simulink model "VMC_14Dof_2024a"  (R2024a)
settings: Solver=FixedStepDiscrete  StartTime=0.0  StopTime=10.0  FixedStep=0.001  RelTol=1e-3
InitFcn:
  | unlinear_14DOF_Parameters
undefined symbols (not defined in the file): Bf, Br, Cp_fl, Cp_fr, Cp_rl, Cp_rr, Cs_f, eta_FMotor, eta_RMotor, f, g, He, Hp, i_fa, i_ra, i_sw, I_tire, Ix, Iy, Iz, ks_f, kw, Lf, Lr, m, mb, mu, mw, r, Sampletime, Standstill_buffer, vx0, vxlim, w0
libraries: simulink x32, slpidlib x6
(part 1 of 5)
settings Model: Creator=Technic  LastModifiedBy=Technic
settings SolverCC: ZeroCrossControl=EnableAll
settings OptimizationCC: DefaultParameterBehavior=Inlined  DefaultUnderspecifiedDataType=single  EnhancedBackFolding=on  PassReuseOutputArgsAs=Individual arguments  ZeroExternalMemoryAtStartup=off  ZeroInternalMemoryAtStartup=off  OptimizeBlockOrder=speed  DifferentSizesBufferReuse=on  OptimizationCustomize=off  EfficientTunableParamExpr=on
settings DebuggingCC: AlgebraicLoopMsg=error  BlockPriorityViolationMsg=error  SolverPrmCheckMsg=error  ParameterPrecisionLossMsg=none  ParamPrecisionLossAbsoluteDiffThreshold=1e-12  ParamPrecisionLossRelativeDiffThreshold=1e-10  ParameterTunabilityLossMsg=error  UnnecessaryDatatypeConvMsg=warning  StateNameClashWarn=warning  AllowedUnitSystems=SI,SI (extended)  AllowAutomaticUnitConversions=off
settings HardwareCC: ProdBitPerPointer=32  ProdBitPerSizeT=32  ProdBitPerPtrDiffT=32  ProdLargestAtomicInteger=Long  ProdLargestAtomicFloat=Double  ProdWordSize=32  ProdHWDeviceType=NXP->Cortex-M4
settings SFSimCC: MATLABDynamicMemAlloc=off
settings RTWCC: Description=Embedded Coder  SystemTargetFile=ert.tlc  GenCodeOnly=on  TemplateMakefile=ert_default_tmf  GenerateReport=on  LaunchReport=on
settings CodeAppCC: ForceParamTrailComments=on  IgnoreCustomStorageClasses=off  OperatorAnnotations=on  SimulinkDataObjDesc=on  SFDataObjDesc=on  InsertBlockDesc=on
settings ERTTargetCC: TargetLangStandard=C99 (ISO)  GenerateSampleERTMain=on  InlinedParameterPlacement=NonHierarchical  ERTCustomFileTemplate=example_file_process.tlc

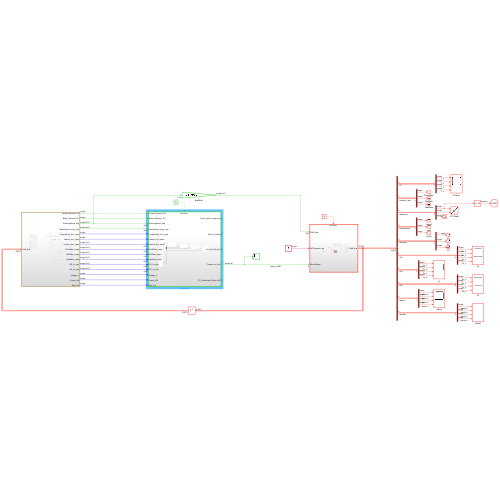
[thumbnail: Simulink's stored preview of the top-level diagram]
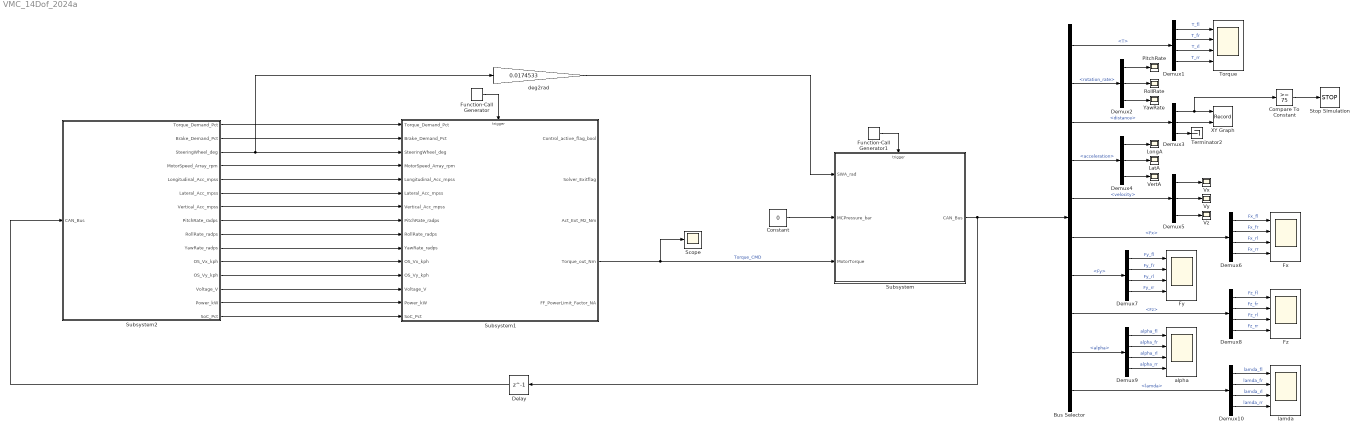
== system VMC_14Dof_2024a ==
  Bus Selector : BusSelector  OutputSignals=T,VehFdbk.rotation_rate,VehFdbk.distance,VehFdbk.acceleration,VehFdbk.velocity,Fx,Fy,Fz,alpha,lamda
  Compare To Constant : simulink/Logic and Bit Operations/Compare To Constant  relop=>=  const=75  OutDataTypeStr=boolean
  Constant : Constant  Value=0  OutDataTypeStr=single
  Delay : Delay  DelayLength=1  InputProcessing=Columns as channels (frame based)
  Demux{1,6..10} (6 alike) : Demux
  Demux{2..5} (4 alike) : Demux  Outputs=3
  Function-Call Generator : simulink/Ports & Subsystems/Function-Call Generator  sample_time=0.005  numberOfIterations=1  DisallowWideOutput=off
  Function-Call Generator1 : simulink/Ports & Subsystems/Function-Call Generator  sample_time=0.001  numberOfIterations=1  DisallowWideOutput=off
  Fx : Scope  NumInputPorts=4
  Fy : Scope  NumInputPorts=4
  Fz : Scope  NumInputPorts=4
  LatA : Scope
  LongA : Scope
  PitchRate : Scope
  RollRate : Scope
  Scope : Scope
  Stop Simulation : Stop
  Subsystem : Subsystem
  Subsystem1 : Subsystem
  Subsystem2 : Subsystem
  Terminator2 : Terminator
  Torque : Scope  NumInputPorts=4
  VertA : Scope
  Vx : Scope
  Vy : Scope
  Vz : Scope
  XY Graph : Record  FileSettingsInternal="{\"entries\":[{\"content\":{\"excelSettings\":{\"content\":{},\"type\":\"Streamout.ExcelSettings\"}},\"type\":\"Streamout.FileSettingStorage\",\"uuid\":\"\"}],\"packageUris\":[\"http:\\/\\/schema.mathworks.com\\/mf0\\/streamout_blocks\\/R2020a\"],\"version\":\"1.0\"}"  Layout=[1 1]  SignalsInternal="{\"entries\":[{\"content\":{\"signals\":[{\"content\":{\"blockPath\":[],\"dimensions\":[1],\"domain\":\"\",\"lineColor\":\"#a2142f\",\"plots\":[ 1 ],\"port\":1,\"signalID\":1,\"signalName\":\"Demux3:1\"},\"type\":\"RecordBlkView.Signal\",\"uuid\":\"\"},{\"content\":{\"blockPath\":[],\"dimensions\":[1],\"domain\":\"\",\"lineColor\":\"#139fff\",\"plots\":[ 1 ],\"port\":2,\"signalID\":2,\"signalName\":\"Demux3:2\"},\"type\":\"RecordBlkView.Signal\",\"uuid\":\"\"}]},\"type\":\"RecordBlkView.InputSignals\",\"uuid\":\"\"}],\"packageUris\":[\"http:\\/\\/schema.mathworks.com\\/mf0\\/streamout_blocks\\/R2020a\"],\"version\":\"1.0\"}"  VisualizationBindings="{\"xyplotplugin\":{\"info\":[{\"series\":[{\"bindingParametersList\":[{\"parameter\":\"X-Axis\",\"signalID\":1,\"signalName\":\"Demux3:1\"},{\"parameter\":\"Y-Axis\",\"signalID\":2,\"signalName\":\"Demux3:2\"}],\"seriesID\":0}],\"subplotID\":1}]}}"  CompatibilityTag=XY  st=-1
  YawRate : Scope
  alpha : Scope  NumInputPorts=4
  deg2rad : Gain  Gain=0.0174533
  lamda : Scope  NumInputPorts=4
  wires:
  Function-Call Generator/1 -> Subsystem1/Trigger
  Subsystem2/3(SteeringWheel_deg) -> deg2rad/1, Subsystem1/3(SteeringWheel_deg)
  Constant/1 -> Subsystem/2(MCPressure_bar)
  Subsystem1/4(Torque_out_Nm) -> Scope/1, Subsystem/3(MotorTorque)  "Torque_CMD"
  Function-Call Generator1/1 -> Subsystem/Trigger
  Subsystem2/1(Torque_Demand_Pct) -> Subsystem1/1(Torque_Demand_Pct)
  Subsystem2/2(Brake_Demand_Pct) -> Subsystem1/2(Brake_Demand_Pct)
  Subsystem2/4(MotorSpeed_Array_rpm) -> Subsystem1/4(MotorSpeed_Array_rpm)
  Subsystem2/5(Longitudinal_Acc_mpss) -> Subsystem1/5(Longitudinal_Acc_mpss)
  Subsystem2/6(Lateral_Acc_mpss) -> Subsystem1/6(Lateral_Acc_mpss)
  Subsystem2/7(Vertical_Acc_mpss) -> Subsystem1/7(Vertical_Acc_mpss)
  Subsystem2/8(PitchRate_radps) -> Subsystem1/8(PitchRate_radps)
  Subsystem2/9(RollRate_radps) -> Subsystem1/9(RollRate_radps)
  Subsystem2/10(YawRate_radps) -> Subsystem1/10(YawRate_radps)
  Subsystem2/11(OS_Vx_kph) -> Subsystem1/11(OS_Vx_kph)
  Subsystem2/12(OS_Vy_kph) -> Subsystem1/12(OS_Vy_kph)
  Subsystem2/13(Voltage_V) -> Subsystem1/13(Voltage_V)
  Subsystem2/14(Power_kW) -> Subsystem1/14(Power_kW)
  Subsystem2/15(SoC_Pct) -> Subsystem1/15(SoC_Pct)
  deg2rad/1 -> Subsystem/1(SWA_rad)
  Delay/1 -> Subsystem2/1(CAN_Bus)
  Demux8/2 -> Fz/2  "Fz_fr"
  Demux9/3 -> alpha/3  "alpha_rl"
  Demux1/3 -> Torque/3  "T_rl"
  Demux2/2 -> RollRate/1
  Demux6/4 -> Fx/4  "Fx_rr"
  Demux10/3 -> lamda/3  "lamda_rl"
  Demux4/3 -> VertA/1
  Demux7/2 -> Fy/2  "Fy_fr"
  Demux9/4 -> alpha/4  "alpha_rr"
  Bus Selector/9 -> Demux9/1  "<alpha>"
  Demux10/4 -> lamda/4  "lamda_rr"
  Demux8/4 -> Fz/4  "Fz_rr"
  Demux1/2 -> Torque/2  "T_fr"
  Demux5/3 -> Vz/1
  Demux4/2 -> LatA/1
  Bus Selector/7 -> Demux7/1  "<Fy>"
  Demux6/3 -> Fx/3  "Fx_rl"
  Demux3/3 -> Terminator2/1
  Bus Selector/4 -> Demux4/1  "<acceleration>"
  Bus Selector/6 -> Demux6/1  "<Fx>"
  Demux3/2 -> XY Graph/2
  Demux1/4 -> Torque/4  "T_rr"
  Bus Selector/3 -> Demux3/1  "<distance>"
  Demux9/2 -> alpha/2  "alpha_fr"
  Demux1/1 -> Torque/1  "T_fl"
  Demux8/3 -> Fz/3  "Fz_rl"
  Subsystem/1(CAN_Bus) -> Delay/1, Bus Selector/1
  Bus Selector/5 -> Demux5/1  "<velocity>"
  Demux8/1 -> Fz/1  "Fz_fl"
  Demux3/1 -> Compare To Constant/1, XY Graph/1
  Demux7/4 -> Fy/4  "Fy_rr"
  Demux5/1 -> Vx/1
  Compare To Constant/1 -> Stop Simulation/1
  Demux9/1 -> alpha/1  "alpha_fl"
  Bus Selector/10 -> Demux10/1  "<lamda>"
  Demux10/1 -> lamda/1  "lamda_fl"
  Demux7/1 -> Fy/1  "Fy_fl"
  Demux7/3 -> Fy/3  "Fy_rl"
  Demux5/2 -> Vy/1
  Demux2/1 -> PitchRate/1
  Demux6/1 -> Fx/1  "Fx_fl"
  Bus Selector/2 -> Demux2/1  "<rotation_rate>"
  Bus Selector/8 -> Demux8/1  "<Fz>"
  Demux10/2 -> lamda/2  "lamda_fr"
  Demux6/2 -> Fx/2  "Fx_fr"
  Demux2/3 -> YawRate/1
  Demux4/1 -> LongA/1
  Bus Selector/1 -> Demux1/1  "<T>"

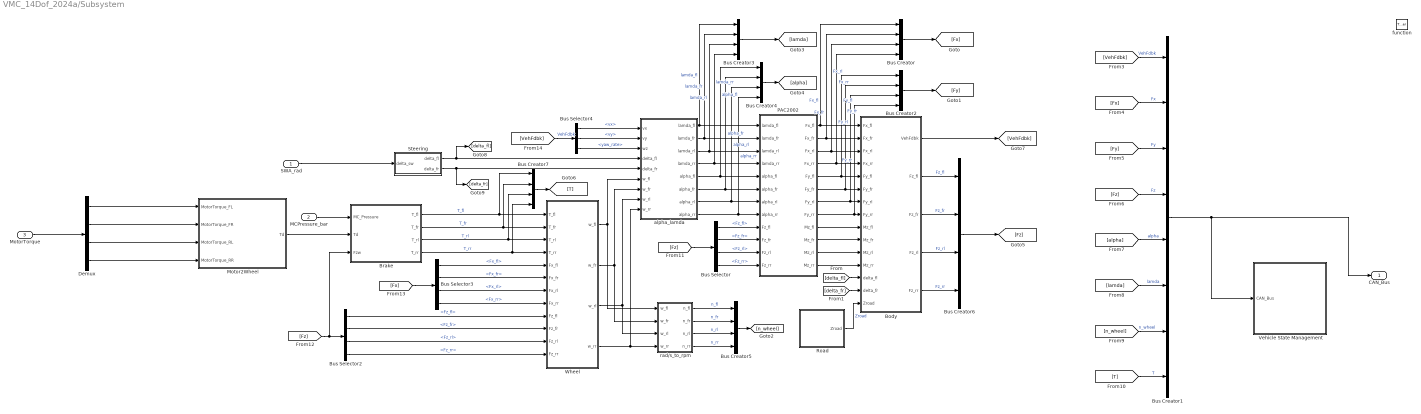
== system VMC_14Dof_2024a/Subsystem ==
  SWA_rad : Inport
  MCPressure_bar : Inport  Port=2
  MotorTorque : Inport  Port=3
  function : TriggerPort  TriggerType=function-call  VariantControl=(inherit)
  Body : Subsystem
  Brake : Subsystem
  Bus Creator{,2..7} (7 alike) : BusCreator  Inputs=4
  Bus Creator1 : BusCreator  Inputs=8
  Bus Selector : BusSelector  OutputSignals=Fz_fl,Fz_fr,Fz_rl,Fz_rr
  Bus Selector2 : BusSelector  OutputSignals=Fz_fl,Fz_fr,Fz_rl,Fz_rr
  Bus Selector3 : BusSelector  OutputSignals=Fx_fl,Fx_fr,Fx_rl,Fx_rr
  Bus Selector4 : BusSelector  OutputSignals=velocity.vx,velocity.vy,rotation_rate.yaw_rate
  Demux : Demux
  Motor2Wheel : Subsystem
  PAC2002 : Subsystem
  Road : Subsystem
  Steering : Subsystem
  Vehicle State Management : Subsystem
  Wheel : Subsystem
  alpha_lamda : Subsystem
  rad/s_to_rpm : Subsystem
  CAN_Bus : Outport  VectorParamsAs1DForOutWhenUnconnected=off
  wires:
  Demux/4 -> Motor2Wheel/4(MotorTorque_RR)
  Brake/2(T_fr) -> Wheel/2(T_fr), Bus Creator7/2  "T_fr"
  Brake/4(T_rr) -> Wheel/4(T_rr), Bus Creator7/4  "T_rr"
  PAC2002/9(Mz_fl) -> Body/9(Mz_fl)
  Bus Creator1/1 -> CAN_Bus/1, Vehicle State Management/1(CAN_Bus)
  Brake/3(T_rl) -> Wheel/3(T_rl), Bus Creator7/3  "T_rl"
  [VehFdbk] -> Bus Selector4/1  "VehFdbk"
  MCPressure_bar/1 -> Brake/1(MC_Pressure)
  [alpha] -> Bus Creator1/5  "alpha"
  Demux/3 -> Motor2Wheel/3(MotorTorque_RL)
  PAC2002/3(Fx_rl) -> Body/3(Fx_rl), Bus Creator/3  "Fx_rl"
  PAC2002/10(Mz_fr) -> Body/10(Mz_fr)
  Wheel/3(w_rl) -> alpha_lamda/8(w_rl), rad/s_to_rpm/3(w_rl)
  alpha_lamda/5(alpha_fl) -> Bus Creator4/1, PAC2002/5(alpha_fl)  "alpha_fl"
  Bus Creator3/1 -> [lamda]
  Bus Selector3/1 -> Wheel/5(Fx_fl)  "<Fx_fl>"
  Wheel/2(w_fr) -> alpha_lamda/7(w_fr), rad/s_to_rpm/2(w_fr)
  Steering/2(delta_fr) -> alpha_lamda/5(delta_fr), [delta_fr]
  Bus Selector2/1 -> Wheel/9(Fz_fl)  "<Fz_fl>"
  PAC2002/4(Fx_rr) -> Body/4(Fx_rr), Bus Creator/4  "Fx_rr"
  Bus Selector/2 -> PAC2002/10(Fz_fr)  "<Fz_fr>"
  Wheel/1(w_fl) -> alpha_lamda/6(w_fl), rad/s_to_rpm/1(w_fl)
  [Fx] -> Bus Selector3/1
  [T] -> Bus Creator1/8  "T"
  [Fz] -> Bus Creator1/4  "Fz"
  Body/2(Fz_fl) -> Bus Creator6/1  "Fz_fl"
  Bus Selector3/2 -> Wheel/6(Fx_fr)  "<Fx_fr>"
  Bus Selector2/3 -> Wheel/11(Fz_rl)  "<Fz_rl>"
  PAC2002/12(Mz_rr) -> Body/12(Mz_rr)
  Bus Creator2/1 -> [Fy]
  [VehFdbk] -> Bus Creator1/1  "VehFdbk"
  alpha_lamda/8(alpha_rr) -> Bus Creator4/4, PAC2002/8(alpha_rr)  "alpha_rr"
  PAC2002/2(Fx_fr) -> Body/2(Fx_fr), Bus Creator/2  "Fx_fr"
  Bus Selector2/2 -> Wheel/10(Fz_fr)  "<Fz_fr>"
  Bus Selector/4 -> PAC2002/12(Fz_rr)  "<Fz_rr>"
  [Fx] -> Bus Creator1/2  "Fx"
  rad/s_to_rpm/2(n_fr) -> Bus Creator5/2  "n_fr"
  Body/5(Fz_rr) -> Bus Creator6/4  "Fz_rr"
  alpha_lamda/3(lamda_rl) -> Bus Creator3/3, PAC2002/3(lamda_rl)  "lamda_rl"
  Bus Selector3/3 -> Wheel/7(Fx_rl)  "<Fx_rl>"
  Bus Selector/1 -> PAC2002/9(Fz_fl)  "<Fz_fl>"
  [n_wheel] -> Bus Creator1/7  "n_wheel"
  Bus Creator7/1 -> [T]
  [Fz] -> Brake/3(Fzw), Bus Selector2/1
  Body/3(Fz_fr) -> Bus Creator6/2  "Fz_fr"
  alpha_lamda/7(alpha_rl) -> Bus Creator4/3, PAC2002/7(alpha_rl)  "alpha_rl"
  [Fz] -> Bus Selector/1
  PAC2002/6(Fy_fr) -> Bus Creator2/2, Body/6(Fy_fr)  "Fy_fr"
  [delta_fl] -> Body/13(delta_fl)
  Bus Selector/3 -> PAC2002/11(Fz_rl)  "<Fz_rl>"
  Bus Selector3/4 -> Wheel/8(Fx_rr)  "<Fx_rr>"
  rad/s_to_rpm/4(n_rr) -> Bus Creator5/4  "n_rr"
  SWA_rad/1 -> Steering/1(delta_sw)
  Bus Selector4/3 -> alpha_lamda/3(wz)  "<yaw_rate>"
  [Fy] -> Bus Creator1/3  "Fy"
  MotorTorque/1 -> Demux/1
  alpha_lamda/1(lamda_fl) -> Bus Creator3/1, PAC2002/1(lamda_fl)  "lamda_fl"
  PAC2002/7(Fy_rl) -> Bus Creator2/3, Body/7(Fy_rl)  "Fy_rl"
  Road/1(Zroad) -> Body/15(Zroad)  "Zroad"
  [delta_fr] -> Body/14(delta_fr)
  Bus Creator6/1 -> [Fz]
  PAC2002/1(Fx_fl) -> Body/1(Fx_fl), Bus Creator/1  "Fx_fl"
  alpha_lamda/6(alpha_fr) -> Bus Creator4/2, PAC2002/6(alpha_fr)  "alpha_fr"
  Wheel/4(w_rr) -> alpha_lamda/9(w_rr), rad/s_to_rpm/4(w_rr)
  Motor2Wheel/1(Td) -> Brake/2(Td)
  Bus Creator4/1 -> [alpha]
  Bus Selector2/4 -> Wheel/12(Fz_rr)  "<Fz_rr>"
  alpha_lamda/2(lamda_fr) -> Bus Creator3/2, PAC2002/2(lamda_fr)  "lamda_fr"
  PAC2002/5(Fy_fl) -> Bus Creator2/1, Body/5(Fy_fl)  "Fy_fl"
  Demux/2 -> Motor2Wheel/2(MotorTorque_FR)
  Bus Creator5/1 -> [n_wheel]
  PAC2002/11(Mz_rl) -> Body/11(Mz_rl)
  Body/1(VehFdbk) -> [VehFdbk]
  alpha_lamda/4(lamda_rr) -> Bus Creator3/4, PAC2002/4(lamda_rr)  "lamda_rr"
  Bus Selector4/2 -> alpha_lamda/2(vy)  "<vy>"
  Demux/1 -> Motor2Wheel/1(MotorTorque_FL)
  PAC2002/8(Fy_rr) -> Bus Creator2/4, Body/8(Fy_rr)  "Fy_rr"
  rad/s_to_rpm/1(n_fl) -> Bus Creator5/1  "n_fl"
  rad/s_to_rpm/3(n_rl) -> Bus Creator5/3  "n_rl"
  Steering/1(delta_fl) -> alpha_lamda/4(delta_fl), [delta_fl]
  Bus Selector4/1 -> alpha_lamda/1(vx)  "<vx>"
  [lamda] -> Bus Creator1/6  "lamda"
  Bus Creator/1 -> [Fx]
  Brake/1(T_fl) -> Wheel/1(T_fl), Bus Creator7/1  "T_fl"
  Body/4(Fz_rl) -> Bus Creator6/3  "Fz_rl"

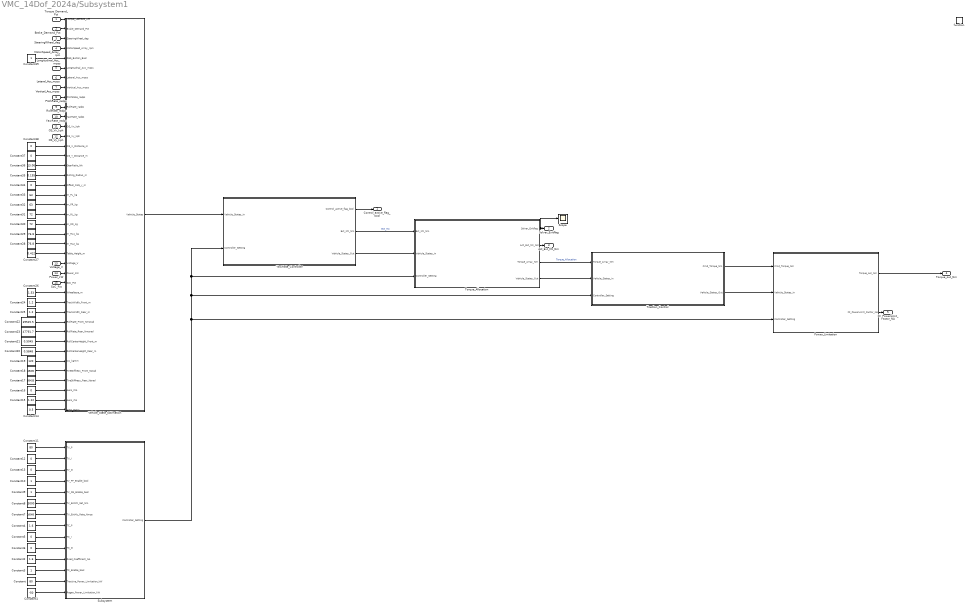
== system VMC_14Dof_2024a/Subsystem1 ==
  Torque_Demand_Pct : Inport
  Brake_Demand_Pct : Inport  Port=2
  SteeringWheel_deg : Inport  Port=3
  MotorSpeed_Array_rpm : Inport  Port=4
  Longitudinal_Acc_mpss : Inport  Port=5
  Lateral_Acc_mpss : Inport  Port=6
  Vertical_Acc_mpss : Inport  Port=7
  PitchRate_radps : Inport  Port=8
  RollRate_radps : Inport  Port=9
  YawRate_radps : Inport  Port=10
  OS_Vx_kph : Inport  Port=11
  OS_Vy_kph : Inport  Port=12
  Voltage_V : Inport  Port=13
  Power_kW : Inport  Port=14
  SoC_Pct : Inport  Port=15
  function : TriggerPort  TriggerType=function-call  VariantControl=(inherit)
  Constant : Constant  Value=80  OutDataTypeStr=single
  Constant1 : Constant  Value=-50  OutDataTypeStr=single
  Constant{3,9..10,39} (4 alike) : Constant  OutDataTypeStr=boolean
  Constant11 : Constant  Value=80  OutDataTypeStr=single
  Constant{5..6,12..13,16,34,37..38} (8 alike) : Constant  Value=0  OutDataTypeStr=single
  Constant14 : Constant  Value=0.5  OutDataTypeStr=single
  Constant15 : Constant  Value=1.22  OutDataTypeStr=single
  Constant17 : Constant  Value=50433  OutDataTypeStr=single
  Constant18 : Constant  Value=48482  OutDataTypeStr=single
  Constant19 : Constant  Value=120  OutDataTypeStr=single
  Constant2 : Constant  Value=1.6  OutDataTypeStr=single
  Constant20 : Constant  Value=0.5848  OutDataTypeStr=single
  Constant21 : Constant  Value=0.5045  OutDataTypeStr=single
  Constant22 : Constant  Value=39525.5  OutDataTypeStr=single
  Constant23 : Constant  Value=47791.7  OutDataTypeStr=single
  Constant24 : Constant  Value=1.2  OutDataTypeStr=single
  Constant25 : Constant  Value=1.2  OutDataTypeStr=single
  Constant26 : Constant  Value=1.53  OutDataTypeStr=single
  Constant27 : Constant  Value=0.412  OutDataTypeStr=single
  Constant28 : Constant  Value=76.8  OutDataTypeStr=single
  Constant29 : Constant  Value=76.8  OutDataTypeStr=single
  Constant30 : Constant  Value=72  OutDataTypeStr=single
  Constant31 : Constant  Value=72  OutDataTypeStr=single
  Constant32 : Constant  Value=63  OutDataTypeStr=single
  Constant33 : Constant  Value=63  OutDataTypeStr=single
  Constant35 : Constant  Value=0.195  OutDataTypeStr=single
  Constant36 : Constant  Value=13.06  OutDataTypeStr=single
  Constant4 : Constant  Value=1.6  OutDataTypeStr=single
  Constant7 : Constant  Value=10000  OutDataTypeStr=single
  Constant8 : Constant  Value=3000  OutDataTypeStr=single
  Power_Limitation : Subsystem
  Scope : Scope
  Subsystem : Subsystem
  Torque_Allocation : Subsystem  TreatAsAtomicUnit=on  RTWFcnName=Torque_Allocation
      settings: RTWSystemCode=Nonreusable function  RTWFcnNameOpts=User specified
  Traction_Control : Subsystem
  Vehicle_State_Estimation : Subsystem
  YawRate_Controller : Subsystem
  Control_active_flag_bool : Outport
  Solver_Exitflag : Outport  Port=2
  Act_Ext_Mz_Nm : Outport  Port=3
  Torque_out_Nm : Outport  Port=4
  FF_PowerLimit_Factor_NA : Outport  Port=5
  wires:
  Power_Limitation/2(FF_PowerLimit_Factor_NA) -> FF_PowerLimit_Factor_NA/1
  Constant36/1 -> Vehicle_State_Estimation/16(GearRatio_NA)
  Constant31/1 -> Vehicle_State_Estimation/21(m_RL_kg)
  Constant9/1 -> Subsystem/5(TV_FB_Enable_bool)
  Constant25/1 -> Vehicle_State_Estimation/31(TrackWidth_Rear_m)
  YawRate_radps/1 -> Vehicle_State_Estimation/11(YawRate_radps)
  Constant11/1 -> Subsystem/1(TV_P)
  Constant34/1 -> Vehicle_State_Estimation/18(Offset_CoG_y_m)
  Constant30/1 -> Vehicle_State_Estimation/22(m_RR_kg)
  Constant5/1 -> Subsystem/9(TC_I)
  YawRate_Controller/3(Vehicle_States_Out) -> Torque_Allocation/2(Vehicle_States_In)
  Constant1/1 -> Subsystem/14(Regen_Power_Limitation_kW)
  Constant7/1 -> Subsystem/7(TV_ExtMz_Rate_Nmps)
  Subsystem/1(Controller_Setting) -> Torque_Allocation/3(Controller_Setting), YawRate_Controller/2(Controller_Setting), Traction_Control/3(Controller_Setting), Power_Limitation/3(Controller_Setting)
  SteeringWheel_deg/1 -> Vehicle_State_Estimation/3(SteeringWheel_deg)
  Traction_Control/2(Vehicle_States_Out) -> Power_Limitation/2(Vehicle_States_In)
  Power_Limitation/1(Torque_out_Nm) -> Torque_out_Nm/1
  Constant35/1 -> Vehicle_State_Estimation/17(Rolling_Radius_m)
  RollRate_radps/1 -> Vehicle_State_Estimation/10(RollRate_radps)
  Constant10/1 -> Subsystem/4(TV_FF_Enable_bool)
  Constant6/1 -> Subsystem/10(TC_D)
  Lateral_Acc_mpss/1 -> Vehicle_State_Estimation/7(Lateral_Acc_mpss)
  PitchRate_radps/1 -> Vehicle_State_Estimation/9(PitchRate_radps)
  Torque_Allocation/3(Torque_Array_Nm) -> Traction_Control/1(Torque_Array_Nm)  "Torque_Allocation"
  Torque_Allocation/4(Vehicle_States_Out) -> Traction_Control/2(Vehicle_States_In)
  Constant28/1 -> Vehicle_State_Estimation/24(m_RL2_kg)
  Constant23/1 -> Vehicle_State_Estimation/33(RollRate_Rear_Nmprad)
  Longitudinal_Acc_mpss/1 -> Vehicle_State_Estimation/6(Longitudinal_Acc_mpss)
  Constant2/1 -> Subsystem/11(Road_Coefficient_NA)
  YawRate_Controller/2(Ext_Mz_Nm) -> Torque_Allocation/1(Ext_Mz_Nm)  "Ext_Mz"
  Constant38/1 -> Vehicle_State_Estimation/14(OS_X_Distance_m)
  MotorSpeed_Array_rpm/1 -> Vehicle_State_Estimation/4(MotorSpeed_Array_rpm)
  Constant26/1 -> Vehicle_State_Estimation/29(Wheelbase_m)
  Constant18/1 -> Vehicle_State_Estimation/37(TireStiffness_Front_Nprad)
  Constant22/1 -> Vehicle_State_Estimation/32(RollRate_Front_Nmprad)
  Traction_Control/1(Cmd_Torque_Nm) -> Power_Limitation/1(Cmd_Torque_Nm)
  Constant16/1 -> Vehicle_State_Estimation/39(Aero_ClA)
  OS_Vx_kph/1 -> Vehicle_State_Estimation/12(OS_Vx_kph)
  Constant12/1 -> Subsystem/2(TV_I)
  Brake_Demand_Pct/1 -> Vehicle_State_Estimation/2(Brake_Demand_Pct)
  Constant39/1 -> Vehicle_State_Estimation/5(REG_Button_Bool)
  Constant32/1 -> Vehicle_State_Estimation/20(m_FR_kg)
  Constant4/1 -> Subsystem/8(TC_P)
  Constant21/1 -> Vehicle_State_Estimation/34(RollCenterHeight_Front_m)
  Power_kW/1 -> Vehicle_State_Estimation/27(Power_kW)
  Constant13/1 -> Subsystem/3(TV_D)
  Constant27/1 -> Vehicle_State_Estimation/25(Table_Height_m)
  Constant33/1 -> Vehicle_State_Estimation/19(m_FL_kg)
  Torque_Demand_Pct/1 -> Vehicle_State_Estimation/1(Torque_Demand_Pct)
  Constant29/1 -> Vehicle_State_Estimation/23(m_RL1_kg)
  Constant3/1 -> Subsystem/12(TC_Enable_bool)
  Constant24/1 -> Vehicle_State_Estimation/30(TrackWidth_Front_m)
  Constant19/1 -> Vehicle_State_Estimation/36(Izz_kgmm)
  Constant20/1 -> Vehicle_State_Estimation/35(RollCenterHeight_Rear_m)
  Vehicle_State_Estimation/1(Vehicle_States) -> YawRate_Controller/1(Vehicle_States_In)
  Constant14/1 -> Vehicle_State_Estimation/41(Aero_Ratio)
  Constant/1 -> Subsystem/13(Tractive_Power_Limitation_kW)
  OS_Vy_kph/1 -> Vehicle_State_Estimation/13(OS_Vy_kph)
  Constant15/1 -> Vehicle_State_Estimation/40(Aero_rho)
  Constant17/1 -> Vehicle_State_Estimation/38(TireStiffness_Rear_Nprad)
  Constant37/1 -> Vehicle_State_Estimation/15(OS_Y_Distance_m)
  Constant8/1 -> Subsystem/6(TV_ExtMz_Sat_Nm)
  Vertical_Acc_mpss/1 -> Vehicle_State_Estimation/8(Vertical_Acc_mpss)
  Voltage_V/1 -> Vehicle_State_Estimation/26(Voltage_V)
  SoC_Pct/1 -> Vehicle_State_Estimation/28(SoC_Pct)
  Torque_Allocation/1(Solver_Exitflag) -> Scope/1, Solver_Exitflag/1
  YawRate_Controller/1(Control_active_flag_bool) -> Control_active_flag_bool/1
  Torque_Allocation/2(Act_Ext_Mz_Nm) -> Act_Ext_Mz_Nm/1

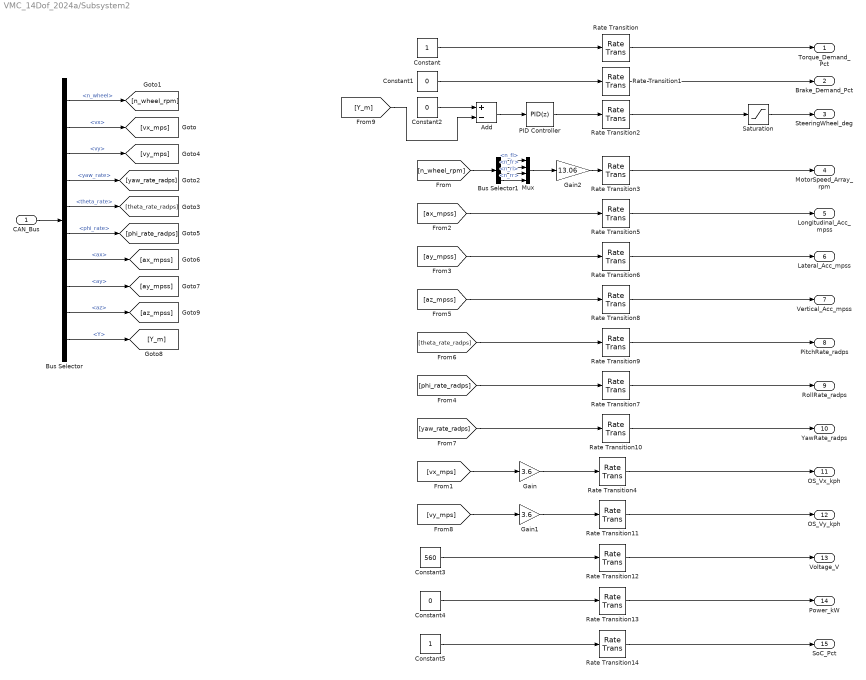
== system VMC_14Dof_2024a/Subsystem2 ==
  CAN_Bus : Inport
  Add : Sum  Inputs=+-
  Bus Selector : BusSelector  OutputSignals=n_wheel,VehFdbk.velocity.vx,VehFdbk.velocity.vy,VehFdbk.rotation_rate.yaw_rate,VehFdbk.rotation_rate.theta_rate,VehFdbk.rotation_rate.phi_rate,VehFdbk.acceleration.ax,VehFdbk.acceleration.ay,VehFdbk.acceleration.az,VehFdbk.distance.Y
  Bus Selector1 : BusSelector  OutputSignals=n_fl,n_fr,n_rl,n_rr
  Constant : Constant  OutDataTypeStr=single
  Constant1 : Constant  Value=0  OutDataTypeStr=single
  Constant2 : Constant  Value=0  OutDataTypeStr=single
  Constant3 : Constant  Value=560  OutDataTypeStr=single
  Constant4 : Constant  Value=0  OutDataTypeStr=single
  Constant5 : Constant  OutDataTypeStr=single
  Gain : Gain  Gain=3.6
  Gain1 : Gain  Gain=3.6
  Gain2 : Gain  Gain=13.06
  Mux : Mux
  PID Controller : slpidlib/PID Controller  Controller=PID  Form=Parallel  TimeDomain=Discrete-time  UseExternalTs=off  SampleTime=-1  IntegratorMethod=Forward Euler  FilterMethod=Forward Euler  ControllerParametersSource=internal  P=5  I=0  UseKiTs=off  D=50  UseExternalDerivativeSource=off  N=100  UseFilter=on  TunerSelectOption=Transfer Function Based (PID Tuner App)  InitialConditionSource=internal  InitialConditionForIntegrator=0  InitialConditionForFilter=0  DifferentiatorICPrevScaledInput=0  ExternalReset=none  TrackingMode=off  Kt=1  LimitOutput=off  SatLimitsSource=internal  UpperSaturationLimit=inf  LowerSaturationLimit=-inf  LinearizeAsGain=on  AntiWindupMode=none  Kb=1  LimitIntegrator=off  UpperIntegratorSaturationLimit=inf  LowerIntegratorSaturationLimit=-inf  POutMin=[]  POutMax=[]  IOutMin=[]  IOutMax=[]  DOutMin=[]  DOutMax=[]  NOutMin=[]  NOutMax=[]  SumOutMin=[]  SumOutMax=[]  SaturationOutMin=[]  SaturationOutMax=[]  PParamMin=[]  PParamMax=[]  IParamMin=[]  IParamMax=[]  DParamMin=[]  DParamMax=[]  NParamMin=[]  NParamMax=[]  KbParamMin=[]  KbParamMax=[]  KtParamMin=[]  KtParamMax=[]  KbOutMin=[]  KbOutMax=[]  KtOutMin=[]  KtOutMax=[]  IntegratorOutMin=[]  IntegratorOutMax=[]  FilterOutMin=[]  FilterOutMax=[]  SumI1OutMin=[]  SumI1OutMax=[]  SumI2OutMin=[]  SumI2OutMax=[]  SumI3OutMin=[]  SumI3OutMax=[]  SumI4OutMin=[]  SumI4OutMax=[]  SumDOutMin=[]  SumDOutMax=[]  DifferentiatorOutMin=[]  DifferentiatorOutMax=[]  FilterDiffOutCoefMin=[]  FilterDiffOutCoefMax=[]  ReciprocalOutMin=[]  ReciprocalOutMax=[]  SumDenOutMin=[]  SumDenOutMax=[]  SumNumOutMin=[]  SumNumOutMax=[]  DivideOutMin=[]  DivideOutMax=[]  UdiffTsProdOutMin=[]  UdiffTsProdOutMax=[]  NTsProdOutMin=[]  NTsProdOutMax=[]  UintegralTsProdOutMin=[]  UintegralTsProdOutMax=[]  UngainTsProdOutMin=[]  UngainTsProdOutMax=[]  ClampingZeroOutDataTypeStr=Inherit: Inherit via back propagation  ClampingZeroOutMin=[]  ClampingZeroOutMax=[]  FilterDenConstantOutDataTypeStr=Inherit: Inherit via back propagation  FilterDenConstantOutMin=[]  FilterDenConstantOutMax=[]  PCopyOutDataTypeStr=Inherit: Inherit via back propagation  PCopyOutMin=[]  PCopyOutMax=[]  NCopyOutDataTypeStr=Inherit: Inherit via back propagation  NCopyOutMin=[]  NCopyOutMax=[]  IntegratorContinuousStateAttributes=''  IntegratorStateMustResolveToSignalObject=off  IntegratorRTWStateStorageClass=Auto  FilterContinuousStateAttributes=''  FilterStateMustResolveToSignalObject=off  FilterRTWStateStorageClass=Auto  ParallelPVariant=InternalParameters  IdealPVariant=Disabled  IVariant=InternalParameters  DVariant=InternalParameters  IntegratorVariant=Discrete  SatVariant=Disabled  AWVariant=Passthrough  PCopyVariant=Disabled  TRVariant=Disabled  FdbkBlocksVariant=Forward  IdealPFdbkVariant=Disabled  SatFdbkVariant=Disabled  DerivativeFilterVariant=ForwardEulerFilter  NVariant=InternalParameters  NCopyVariant=Disabled  FilterICVariant=InternalICsFilter  IntegratorICVariant=InternalICs  ExternalResetVariant=Disabled  TRSumVariant=Passthrough  SumFdbkVariant=Disabled  SumVariant=Sum_PID  TsampFilterVariant=InternalTs  TsampNgainVariant=Passthrough  TsampIntegralVariant=Disabled_SignalSpec  ExternalSaturationOutDataTypeStr=Inherit: Same as second input  DerivativeSourceVariant=ErrorSignal
  Rate Transition{,1..3} (4 alike) : RateTransition  OutPortSampleTime=0.005
  Rate Transition{4..11} (8 alike) : RateTransition  OutPortSampleTime=0.02
  Rate Transition12 : RateTransition  OutPortSampleTime=0.01
  Rate Transition13 : RateTransition  OutPortSampleTime=0.01
  Rate Transition14 : RateTransition  OutPortSampleTime=0.01
  Saturation : Saturate  UpperLimit=117  LowerLimit=-117
  Torque_Demand_Pct : Outport
  Brake_Demand_Pct : Outport  Port=2
  SteeringWheel_deg : Outport  Port=3
  MotorSpeed_Array_rpm : Outport  Port=4
  Longitudinal_Acc_mpss : Outport  Port=5
  Lateral_Acc_mpss : Outport  Port=6
  Vertical_Acc_mpss : Outport  Port=7
  PitchRate_radps : Outport  Port=8
  RollRate_radps : Outport  Port=9
  YawRate_radps : Outport  Port=10
  OS_Vx_kph : Outport  Port=11
  OS_Vy_kph : Outport  Port=12
  Voltage_V : Outport  Port=13
  Power_kW : Outport  Port=14
  SoC_Pct : Outport  Port=15
  wires:
  Constant/1 -> Rate Transition/1
  Constant1/1 -> Rate Transition1/1
  Constant2/1 -> Add/1
  CAN_Bus/1 -> Bus Selector/1
  Bus Selector/10 -> [Y_m]  "<Y>"
  Bus Selector/2 -> [vx_mps]  "<vx>"
  Bus Selector/1 -> [n_wheel_rpm]  "<n_wheel>"
  Bus Selector/4 -> [yaw_rate_radps]  "<yaw_rate>"
  Bus Selector/5 -> [theta_rate_radps]  "<theta_rate>"
  Bus Selector/3 -> [vy_mps]  "<vy>"
  Bus Selector/6 -> [phi_rate_radps]  "<phi_rate>"
  Bus Selector/7 -> [ax_mpss]  "<ax>"
  Bus Selector/8 -> [ay_mpss]  "<ay>"
  Bus Selector1/1 -> Mux/1  "<n_fl>"
  Bus Selector1/2 -> Mux/2  "<n_fr>"
  Bus Selector1/3 -> Mux/3  "<n_rl>"
  Bus Selector1/4 -> Mux/4  "<n_rr>"
  Mux/1 -> Gain2/1
  Rate Transition3/1 -> MotorSpeed_Array_rpm/1
  [vx_mps] -> Gain/1
  Gain/1 -> Rate Transition4/1
  Rate Transition4/1 -> OS_Vx_kph/1
  [ax_mpss] -> Rate Transition5/1
  Rate Transition5/1 -> Longitudinal_Acc_mpss/1
  [ay_mpss] -> Rate Transition6/1
  Rate Transition6/1 -> Lateral_Acc_mpss/1
  Bus Selector/9 -> [az_mpss]  "<az>"
  [az_mpss] -> Rate Transition8/1
  Rate Transition8/1 -> Vertical_Acc_mpss/1
  [phi_rate_radps] -> Rate Transition7/1
  [theta_rate_radps] -> Rate Transition9/1
  Rate Transition9/1 -> PitchRate_radps/1
  Rate Transition7/1 -> RollRate_radps/1
  [yaw_rate_radps] -> Rate Transition10/1
  Rate Transition10/1 -> YawRate_radps/1
  Rate Transition11/1 -> OS_Vy_kph/1
  Gain1/1 -> Rate Transition11/1
  [vy_mps] -> Gain1/1
  Rate Transition12/1 -> Voltage_V/1
  Constant3/1 -> Rate Transition12/1
  Constant4/1 -> Rate Transition13/1
  Rate Transition13/1 -> Power_kW/1
  Rate Transition14/1 -> SoC_Pct/1
  Constant5/1 -> Rate Transition14/1
  Rate Transition/1 -> Torque_Demand_Pct/1
  Rate Transition1/1 -> Brake_Demand_Pct/1
  [Y_m] -> Add/2
  Add/1 -> PID Controller/1
  PID Controller/1 -> Rate Transition2/1
  Saturation/1 -> SteeringWheel_deg/1
  Rate Transition2/1 -> Saturation/1
  [n_wheel_rpm] -> Bus Selector1/1
  Gain2/1 -> Rate Transition3/1

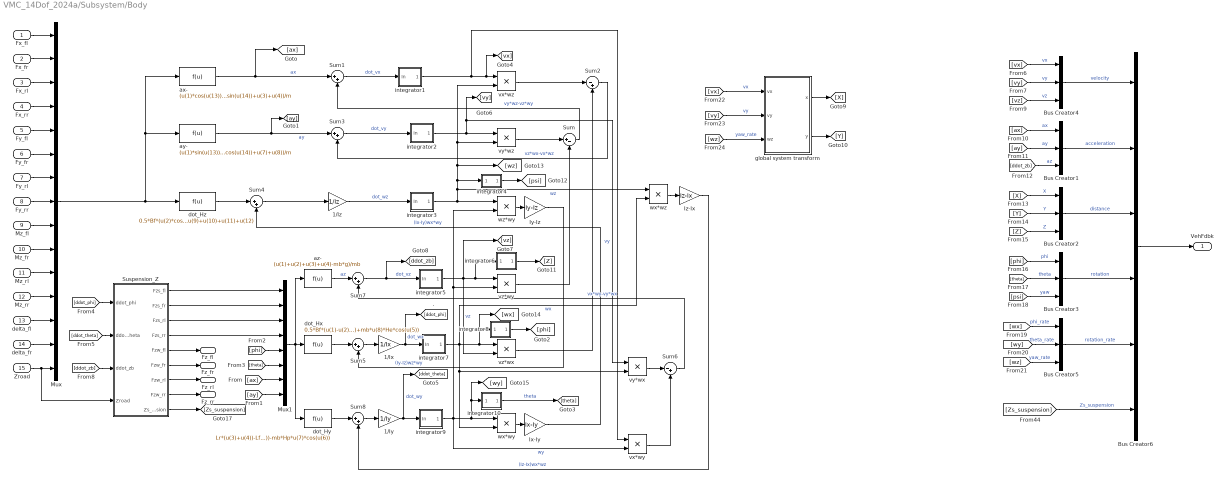
== system VMC_14Dof_2024a/Subsystem/Body ==
  Fx_fl : Inport
  Fx_fr : Inport  Port=2
  Fx_rl : Inport  Port=3
  Fx_rr : Inport  Port=4
  Fy_fl : Inport  Port=5
  Fy_fr : Inport  Port=6
  Fy_rl : Inport  Port=7
  Fy_rr : Inport  Port=8
  Mz_fl : Inport  Port=9
  Mz_fr : Inport  Port=10
  Mz_rl : Inport  Port=11
  Mz_rr : Inport  Port=12
  delta_fl : Inport  Port=13
  delta_fr : Inport  Port=14
  Zroad : Inport  Port=15
  1/Ix : Gain  Gain=1/Ix  OutDataTypeStr=single
  1/Iy : Gain  Gain=1/Iy  OutDataTypeStr=single
  1/Iz : Gain  Gain=1/Iz  OutDataTypeStr=single
  Bus Creator{1..5} (5 alike) : BusCreator  Inputs=3
  Bus Creator6 : BusCreator  Inputs=6
  Ix-Iy : Gain  Gain=Ix-Iy
  Iy-Iz : Gain  Gain=Iy-Iz
  Iz-Ix : Gain  Gain=Iz-Ix
  Mux : Mux  Inputs=15
  Mux1 : Mux  Inputs=8
  Sum : Sum  Inputs=|+-
  Sum1 : Sum  Inputs=|++  OutDataTypeStr=single  AccumDataTypeStr=single
  Sum2 : Sum  Inputs=|-+
  Sum{3..5,8} (4 alike) : Sum  Inputs=|++
  Sum6 : Sum  Inputs=|-+
  Sum7 : Sum  Inputs=|++  OutDataTypeStr=single
  Suspension_Z : Subsystem
  ax- : Fcn  Expr=(u(1)*cos(u(13))+u(2)*cos(u(14))-u(5)*sin(u(13))-u(6)*sin(u(14))+u(3)+u(4))/m
  ay- : Fcn  Expr=(u(1)*sin(u(13))+u(2)*sin(u(14))+u(5)*cos(u(13))+u(6)*cos(u(14))+u(7)+u(8))/m
  az- : Fcn  Expr=(u(1)+u(2)+u(3)+u(4)-mb*g)/mb
  dot_Hx : Fcn  Expr=0.5*Bf*(u(1)-u(2))+0.5*Br*(u(3)-u(4))+mb*g*He*sin(u(5))+mb*u(8)*He*cos(u(5))
  dot_Hy : Fcn  Expr=Lr*(u(3)+u(4))-Lf*(u(1)+u(2))+mb*g*Hp*sin(u(6))-mb*Hp*u(7)*cos(u(6))
  dot_Hz : Fcn  Expr=0.5*Bf*(u(2)*cos(u(14))-u(1)*cos(u(13))-u(6)*sin(u(14))+u(5)*sin(u(13)))+0.5*Br*(u(4)-u(3))+Lf*(u(1)*sin(u(13))+u(5)*cos(u(13))+u(2)*sin(u(14))+u(6)*cos(u(14)))-Lr*(u(7)+u(8))+u(9)+u(10)+u(11)+u(12)
  global system transform : Subsystem
  integrator1 : Subsystem
  integrator10 : Subsystem
  integrator2 : Subsystem
  integrator3 : Subsystem
  integrator4 : Subsystem
  integrator5 : Subsystem
  integrator6 : Subsystem
  integrator7 : Subsystem
  integrator8 : Subsystem
  integrator9 : Subsystem
  vx*wy : Product
  vx*wz : Product
  vy*wx : Product
  vy*wz : Product
  vz*wx : Product
  vz*wy : Product
  wx*wy : Product
  wx*wz : Product
  wz*wy : Product
  VehFdbk : Outport  VectorParamsAs1DForOutWhenUnconnected=off
  Fz_fl : Outport  Port=2  VectorParamsAs1DForOutWhenUnconnected=off
  Fz_fr : Outport  Port=3  VectorParamsAs1DForOutWhenUnconnected=off
  Fz_rl : Outport  Port=4  VectorParamsAs1DForOutWhenUnconnected=off
  Fz_rr : Outport  Port=5  VectorParamsAs1DForOutWhenUnconnected=off
  wires:
  Mux1/1 -> az-/1, dot_Hx/1, dot_Hy/1
  Sum8/1 -> 1/Iy/1
  az-/1 -> Sum7/1  "az"
  dot_Hy/1 -> Sum8/1
  ax-/1 -> [ax], Sum1/1  "ax"
  Suspension_Z/8(Fzw_rr) -> Fz_rr/1
  Suspension_Z/7(Fzw_rl) -> Fz_rl/1
  Suspension_Z/6(Fzw_fr) -> Fz_fr/1
  Suspension_Z/5(Fzw_fl) -> Fz_fl/1
  [ddot_zb] -> Suspension_Z/3(ddot_zb)
  [ddot_theta] -> Suspension_Z/2(ddot_theta)
  [ddot_phi] -> Suspension_Z/1(ddot_phi)
  [phi] -> Mux1/5
  Suspension_Z/2(Fzs_fr) -> Mux1/2
  Suspension_Z/3(Fzs_rl) -> Mux1/3
  Suspension_Z/4(Fzs_rr) -> Mux1/4
  Suspension_Z/1(Fzs_fl) -> Mux1/1
  integrator10/1(Out) -> [theta]  "theta"
  Iz-Ix/1 -> Sum8/2  "(Iz-Ix)wx*wz"
  wx*wz/1 -> Iz-Ix/1
  Sum5/1 -> 1/Ix/1
  Iy-Iz/1 -> Sum5/2  "(Iy-Iz)wz*wy"
  dot_Hx/1 -> Sum5/1
  Sum6/1 -> Sum7/2  "vx*wy-vy*wx"
  vx*wy/1 -> Sum6/2
  vy*wx/1 -> Sum6/1
  Sum4/1 -> 1/Iz/1
  dot_Hz/1 -> Sum4/1
  Ix-Iy/1 -> Sum4/2  "(Ix-Iy)wx*wy"
  wx*wy/1 -> Ix-Iy/1
  Sum2/1 -> Sum3/2  "vz*wx-vx*wz"
  vz*wx/1 -> Sum2/2
  vx*wz/1 -> Sum2/1
  Sum/1 -> Sum1/2  "vy*wz-vz*wy"
  vz*wy/1 -> Sum/2
  wz*wy/1 -> Iy-Iz/1
  vy*wz/1 -> Sum/1
  ay-/1 -> [ay], Sum3/1  "ay"
  integrator9/1(Out) -> wx*wy/1, integrator10/1(In), [wy], wz*wy/2, vz*wy/2, vx*wy/2  "wy"
  1/Iy/1 -> integrator9/1(In), [ddot_theta]  "dot_wy"
  1/Ix/1 -> integrator7/1(In), [ddot_phi]  "dot_wx"
  integrator7/1(Out) -> integrator8/1(In), [wx], vz*wx/1, wx*wy/2, vy*wx/2, wx*wz/2  "wx"
  integrator5/1(Out) -> [vz], integrator6/1(In), vz*wy/1, vz*wx/2  "vz"
  Sum7/1 -> integrator5/1(In), [ddot_zb]  "dot_vz"
  integrator3/1(Out) -> wz*wy/1, [wz], vx*wz/2, vy*wz/2, integrator4/1(In), wx*wz/1  "wz"
  1/Iz/1 -> integrator3/1(In)  "dot_wz"
  Sum3/1 -> integrator2/1(In)  "dot_vy"
  integrator2/1(Out) -> vy*wz/1, [vy], vy*wx/1  "vy"
  integrator1/1(Out) -> vx*wy/1, [vx], vx*wz/1
  Sum1/1 -> integrator1/1(In)  "dot_vx"
  Fx_fl/1 -> Mux/1
  Fx_fr/1 -> Mux/2
  Fx_rl/1 -> Mux/3
  Fx_rr/1 -> Mux/4
  Fy_fl/1 -> Mux/5
  Fy_fr/1 -> Mux/6
  Fy_rl/1 -> Mux/7
  Fy_rr/1 -> Mux/8
  Mz_fl/1 -> Mux/9
  Mz_fr/1 -> Mux/10
  Mz_rl/1 -> Mux/11
  Mz_rr/1 -> Mux/12
  delta_fl/1 -> Mux/13
  delta_fr/1 -> Mux/14
  Mux/1 -> ax-/1, ay-/1, dot_Hz/1
  Zroad/1 -> Suspension_Z/4(Zroad), Mux/15
  [ax] -> Mux1/7
  [ay] -> Mux1/8
  global system transform/1(x) -> [X]
  global system transform/2(y) -> [Y]
  [theta] -> Mux1/6
  [ax] -> Bus Creator1/1  "ax"
  Bus Creator2/1 -> Bus Creator6/3  "distance"
  Bus Creator6/1 -> VehFdbk/1
  Bus Creator5/1 -> Bus Creator6/5  "rotation_rate"
  Bus Creator3/1 -> Bus Creator6/4  "rotation"
  [Y] -> Bus Creator2/2  "Y"
  [Zs_suspension] -> Bus Creator6/6  "Zs_suspension"
  [theta] -> Bus Creator3/2  "theta"
  [wz] -> Bus Creator5/3  "yaw_rate"
  [vx] -> Bus Creator4/1  "vx"
  [vy] -> Bus Creator4/2  "vy"
  [ay] -> Bus Creator1/2  "ay"
  [wy] -> Bus Creator5/2  "theta_rate"
  [ddot_zb] -> Bus Creator1/3  "az"
  [Z] -> Bus Creator2/3  "Z"
  Bus Creator4/1 -> Bus Creator6/1  "velocity"
  [phi] -> Bus Creator3/1  "phi"
  [vz] -> Bus Creator4/3  "vz"
  Bus Creator1/1 -> Bus Creator6/2  "acceleration"
  [wx] -> Bus Creator5/1  "phi_rate"
  [psi] -> Bus Creator3/3  "yaw"
  [X] -> Bus Creator2/1  "X"
  integrator6/1(Out) -> [Z]
  integrator4/1(Out) -> [psi]
  [vx] -> global system transform/1(vx)  "vx"
  [vy] -> global system transform/2(vy)  "vy"
  Suspension_Z/9(Zs_suspension) -> [Zs_suspension]
  [wz] -> global system transform/3(wz)  "yaw_rate"
  integrator8/1(Out) -> [phi]

== system VMC_14Dof_2024a/Subsystem/Brake ==
  MC_Pressure : Inport
  Td : Inport  Port=2
  Fzw : Inport  Port=3
  Add{,1..3} (4 alike) : Sum  Inputs=+-  OutDataTypeStr=single
  Bus Selector1 : BusSelector  OutputSignals=T_fl,T_fr,T_rl,T_rr
  Bus Selector3 : BusSelector  OutputSignals=Tb_fl,Tb_fr,Tb_rl,Tb_rr
  WheelBrakeTorque : Subsystem
  T_fl : Outport
  T_fr : Outport  Port=2
  T_rl : Outport  Port=3
  T_rr : Outport  Port=4
  wires:
  Bus Selector3/2 -> [Tb_fr]  "<Tb_fr>"
  Fzw/1 -> WheelBrakeTorque/3(Fzw)
  Add1/1 -> T_fr/1
  Bus Selector1/2 -> [Td_fr]  "<T_fr>"
  Bus Selector3/3 -> [Tb_rl]  "<Tb_rl>"
  [Tb_fl] -> Add/2  "Tb_fl"
  Bus Selector1/3 -> [Td_rl]  "<T_rl>"
  [Tb_rl] -> Add2/2  "Tb_rl"
  Bus Selector3/1 -> [Tb_fl]  "<Tb_fl>"
  Bus Selector3/4 -> [Tb_rr]  "<Tb_rr>"
  Bus Selector1/1 -> [Td_fl]  "<T_fl>"
  [Tb_rr] -> Add3/2  "Tb_rr"
  Td/1 -> Bus Selector1/1, WheelBrakeTorque/2(Td)
  MC_Pressure/1 -> WheelBrakeTorque/1(TMC)
  Add/1 -> T_fl/1
  WheelBrakeTorque/1(WheelBrakeTorque) -> Bus Selector3/1
  [Td_rl] -> Add2/1
  Bus Selector1/4 -> [Td_rr]  "<T_rr>"
  [Td_rr] -> Add3/1
  Add3/1 -> T_rr/1
  [Td_fr] -> Add1/1
  Add2/1 -> T_rl/1
  [Td_fl] -> Add/1
  [Tb_fr] -> Add1/2  "Tb_fr"

== system VMC_14Dof_2024a/Subsystem/Motor2Wheel ==
  MotorTorque_FL : Inport
  MotorTorque_FR : Inport  Port=2
  MotorTorque_RL : Inport  Port=3
  MotorTorque_RR : Inport  Port=4
  Bus Creator : BusCreator  Inputs=4
  Gain : Gain  Gain=eta_FMotor  OutDataTypeStr=single
  Gain1 : Gain  Gain=eta_RMotor  ParamDataTypeStr=single  OutDataTypeStr=single
  Gain2 : Gain  Gain=i_ra  OutDataTypeStr=single
  Gain3 : Gain  Gain=i_ra  OutDataTypeStr=single
  Gain4 : Gain  Gain=eta_FMotor  OutDataTypeStr=single
  Gain5 : Gain  Gain=i_fa  OutDataTypeStr=single
  Gain6 : Gain  Gain=eta_FMotor  OutDataTypeStr=single
  Gain7 : Gain  Gain=i_fa  OutDataTypeStr=single
  Td : Outport  VectorParamsAs1DForOutWhenUnconnected=off
  wires:
  Gain7/1 -> [Td_fr]  "T_fr"
  Gain5/1 -> [Td_fl]  "T_fl"
  MotorTorque_FL/1 -> Gain/1
  Gain3/1 -> [Td_rr]  "T_rr"
  Gain2/1 -> [Td_rl]  "T_rl"
  MotorTorque_RL/1 -> Gain1/1
  [Td_rr] -> Bus Creator/4
  Bus Creator/1 -> Td/1
  [Td_rl] -> Bus Creator/3
  [Td_fl] -> Bus Creator/1
  [Td_fr] -> Bus Creator/2
  Gain/1 -> Gain5/1
  Gain1/1 -> Gain2/1
  MotorTorque_FR/1 -> Gain4/1
  MotorTorque_RR/1 -> Gain6/1
  Gain6/1 -> Gain3/1
  Gain4/1 -> Gain7/1

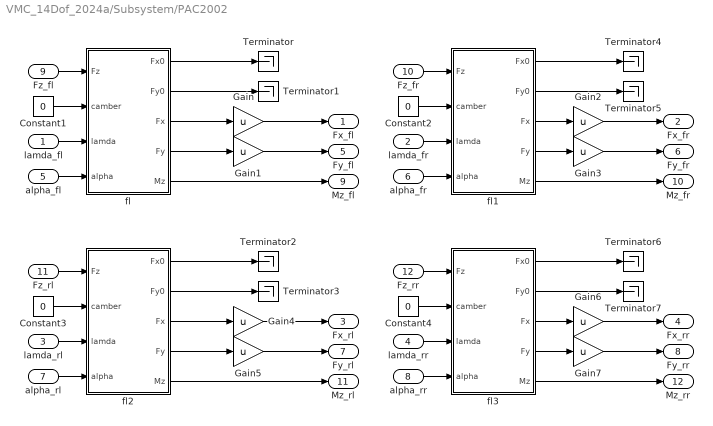
== system VMC_14Dof_2024a/Subsystem/PAC2002 ==
  lamda_fl : Inport
  lamda_fr : Inport  Port=2
  lamda_rl : Inport  Port=3
  lamda_rr : Inport  Port=4
  alpha_fl : Inport  Port=5
  alpha_fr : Inport  Port=6
  alpha_rl : Inport  Port=7
  alpha_rr : Inport  Port=8
  Fz_fl : Inport  Port=9
  Fz_fr : Inport  Port=10
  Fz_rl : Inport  Port=11
  Fz_rr : Inport  Port=12
  Constant{1..4} (4 alike) : Constant  Value=0  OutDataTypeStr=single
  Gain{,1..7} (8 alike) : Gain  Gain=u
  Terminator{,1..7} (8 alike) : Terminator
  fl : MATLAB Function  TreatAsAtomicUnit=on
  fl1 : MATLAB Function  TreatAsAtomicUnit=on
  fl2 : MATLAB Function  TreatAsAtomicUnit=on
  fl3 : MATLAB Function  TreatAsAtomicUnit=on
  Fx_fl : Outport  VectorParamsAs1DForOutWhenUnconnected=off
  Fx_fr : Outport  Port=2  VectorParamsAs1DForOutWhenUnconnected=off
  Fx_rl : Outport  Port=3  VectorParamsAs1DForOutWhenUnconnected=off
  Fx_rr : Outport  Port=4  VectorParamsAs1DForOutWhenUnconnected=off
  Fy_fl : Outport  Port=5  VectorParamsAs1DForOutWhenUnconnected=off
  Fy_fr : Outport  Port=6  VectorParamsAs1DForOutWhenUnconnected=off
  Fy_rl : Outport  Port=7  VectorParamsAs1DForOutWhenUnconnected=off
  Fy_rr : Outport  Port=8  VectorParamsAs1DForOutWhenUnconnected=off
  Mz_fl : Outport  Port=9  VectorParamsAs1DForOutWhenUnconnected=off
  Mz_fr : Outport  Port=10  VectorParamsAs1DForOutWhenUnconnected=off
  Mz_rl : Outport  Port=11  VectorParamsAs1DForOutWhenUnconnected=off
  Mz_rr : Outport  Port=12  VectorParamsAs1DForOutWhenUnconnected=off
  wires:
  Constant4/1 -> fl3/2(camber)
  Constant3/1 -> fl2/2(camber)
  Constant2/1 -> fl1/2(camber)
  Fz_rr/1 -> fl3/1(Fz)
  alpha_rr/1 -> fl3/4(alpha)
  lamda_rr/1 -> fl3/3(lamda)
  Fz_rl/1 -> fl2/1(Fz)
  alpha_rl/1 -> fl2/4(alpha)
  lamda_rl/1 -> fl2/3(lamda)
  Fz_fr/1 -> fl1/1(Fz)
  alpha_fr/1 -> fl1/4(alpha)
  lamda_fr/1 -> fl1/3(lamda)
  Constant1/1 -> fl/2(camber)
  Fz_fl/1 -> fl/1(Fz)
  alpha_fl/1 -> fl/4(alpha)
  lamda_fl/1 -> fl/3(lamda)
  fl/3(Fx) -> Gain/1
  fl/4(Fy) -> Gain1/1
  fl1/4(Fy) -> Gain3/1
  fl3/3(Fx) -> Gain6/1
  fl3/4(Fy) -> Gain7/1
  fl2/3(Fx) -> Gain4/1
  fl2/4(Fy) -> Gain5/1
  fl1/3(Fx) -> Gain2/1
  Gain/1 -> Fx_fl/1
  Gain1/1 -> Fy_fl/1
  Gain2/1 -> Fx_fr/1
  Gain3/1 -> Fy_fr/1
  Gain4/1 -> Fx_rl/1
  Gain5/1 -> Fy_rl/1
  Gain6/1 -> Fx_rr/1
  Gain7/1 -> Fy_rr/1
  fl/1(Fx0) -> Terminator/1
  fl/2(Fy0) -> Terminator1/1
  fl2/1(Fx0) -> Terminator2/1
  fl2/2(Fy0) -> Terminator3/1
  fl1/1(Fx0) -> Terminator4/1
  fl1/2(Fy0) -> Terminator5/1
  fl3/1(Fx0) -> Terminator6/1
  fl3/2(Fy0) -> Terminator7/1
  fl/5(Mz) -> Mz_fl/1
  fl2/5(Mz) -> Mz_rl/1
  fl1/5(Mz) -> Mz_fr/1
  fl3/5(Mz) -> Mz_rr/1

== system VMC_14Dof_2024a/Subsystem/Road ==
  Bus Creator : BusCreator  Inputs=4
  Constant{1..4} (4 alike) : Constant  Value=0  OutDataTypeStr=single
  Zroad : Outport  VectorParamsAs1DForOutWhenUnconnected=off
  wires:
  Constant3/1 -> Bus Creator/4  "Zroad_rr"
  Constant1/1 -> Bus Creator/2  "Zroad_fr"
  Constant2/1 -> Bus Creator/3  "Zroad_rl"
  Bus Creator/1 -> Zroad/1  "Zroad"
  Constant4/1 -> Bus Creator/1  "Zroad_fl"

== system VMC_14Dof_2024a/Subsystem/Steering ==
  delta_sw : Inport
  Add : Sum  OutDataTypeStr=single
  Add2 : Sum  Inputs=-+  OutDataTypeStr=single
  Add3 : Sum  OutDataTypeStr=single
  Constant : Constant  Value=Lr  OutDataTypeStr=single
  Constant1 : Constant  Value=Lf  OutDataTypeStr=single
  Constant2 : Constant  Value=i_sw  OutDataTypeStr=single
  Constant3 : Constant  Value=Br  OutDataTypeStr=single
  Divide : Product  Inputs=*/
  Divide1 : Product  Inputs=/*  OutDataTypeStr=single
  Divide2 : Product  Inputs=/*  OutDataTypeStr=single
  Gain : Gain  Gain=2
  Product : Product  OutDataTypeStr=single
  Product1 : Product
  Trigonometric Function : Trigonometry  Operator=atan
  Trigonometric Function1 : Trigonometry  Operator=tan
  Trigonometric Function2 : Trigonometry  Operator=atan
  delta_fl : Outport  VectorParamsAs1DForOutWhenUnconnected=off
  delta_fr : Outport  Port=2  VectorParamsAs1DForOutWhenUnconnected=off
  wires:
  Constant1/1 -> Add/1
  Constant/1 -> Add/2
  Add/1 -> Gain/1
  delta_sw/1 -> Divide/1
  Constant2/1 -> Divide/2
  Divide/1 -> Trigonometric Function1/1  "delta_s"
  Trigonometric Function1/1 -> Product/1, Product1/2
  Gain/1 -> Product/2, Add3/2, Add2/2
  Constant3/1 -> Product1/1
  Product1/1 -> Add3/1, Add2/1
  Add2/1 -> Divide1/1
  Product/1 -> Divide2/2, Divide1/2
  Divide1/1 -> Trigonometric Function/1
  Trigonometric Function/1 -> delta_fl/1
  Add3/1 -> Divide2/1
  Divide2/1 -> Trigonometric Function2/1
  Trigonometric Function2/1 -> delta_fr/1

== system VMC_14Dof_2024a/Subsystem/Vehicle State Management ==
  CAN_Bus : Inport
  Abs{,1..4} (5 alike) : Abs  SaturateOnIntegerOverflow=off
  Bus Selector : BusSelector  OutputSignals=n_wheel.n_fl,n_wheel.n_fr,n_wheel.n_rl,n_wheel.n_rr,VehFdbk.velocity.vx
  Gain{,1..3} (4 alike) : Gain  Gain=pi/30
  Logical Operator : Logic  Inputs=4  AllPortsSameDT=off  OutDataTypeStr=boolean
  Logical Operator1 : Logic  AllPortsSameDT=off  OutDataTypeStr=boolean
  StandStill_thres : Subsystem
  StandStill_thres1 : Subsystem
  StandStill_thres2 : Subsystem
  StandStill_thres3 : Subsystem
  StandStill_thres4 : Subsystem
  tag scope: StandStill_flag=global
  wires:
  Bus Selector/2 -> Abs1/1  "<n_fr>"
  Bus Selector/1 -> Abs/1  "<n_fl>"
  CAN_Bus/1 -> Bus Selector/1
  Bus Selector/4 -> Abs3/1  "<n_rr>"
  Bus Selector/3 -> Abs2/1  "<n_rl>"
  Abs/1 -> Gain/1
  Abs1/1 -> Gain1/1
  Abs2/1 -> Gain2/1
  Abs3/1 -> Gain3/1
  StandStill_thres/1(Out1) -> Logical Operator/1
  StandStill_thres1/1(Out1) -> Logical Operator/2
  StandStill_thres2/1(Out1) -> Logical Operator/3
  Abs4/1 -> StandStill_thres4/1(In1)
  Logical Operator/1 -> Logical Operator1/1
  StandStill_thres4/1(Out1) -> Logical Operator1/2
  Bus Selector/5 -> Abs4/1  "<vx>"
  Gain/1 -> StandStill_thres/1(In1)
  Gain1/1 -> StandStill_thres1/1(In1)
  Gain2/1 -> StandStill_thres2/1(In1)
  Logical Operator1/1 -> [StandStill_flag]
  StandStill_thres3/1(Out1) -> Logical Operator/4
  Gain3/1 -> StandStill_thres3/1(In1)

== system VMC_14Dof_2024a/Subsystem/Wheel ==
  T_fl : Inport
  T_fr : Inport  Port=2
  T_rl : Inport  Port=3
  T_rr : Inport  Port=4
  Fx_fl : Inport  Port=5
  Fx_fr : Inport  Port=6
  Fx_rl : Inport  Port=7
  Fx_rr : Inport  Port=8
  Fz_fl : Inport  Port=9
  Fz_fr : Inport  Port=10
  Fz_rl : Inport  Port=11
  Fz_rr : Inport  Port=12
  fl : Subsystem
  fr : Subsystem
  rl : Subsystem
  rr : Subsystem
  w_fl : Outport  VectorParamsAs1DForOutWhenUnconnected=off
  w_fr : Outport  Port=2  VectorParamsAs1DForOutWhenUnconnected=off
  w_rl : Outport  Port=3  VectorParamsAs1DForOutWhenUnconnected=off
  w_rr : Outport  Port=4  VectorParamsAs1DForOutWhenUnconnected=off
  wires:
  rr/1(w_rr) -> w_rr/1
  Fz_rr/1 -> rr/3(Fz_rr)
  Fx_rr/1 -> rr/2(Fx_rr)
  T_rr/1 -> rr/1(T_rr)
  rl/1(w_rl) -> w_rl/1
  Fz_rl/1 -> rl/3(Fz_rl)
  Fx_rl/1 -> rl/2(Fx_rl)
  T_rl/1 -> rl/1(T_rl)
  Fz_fr/1 -> fr/3(Fz_fr)
  Fx_fr/1 -> fr/2(Fx_fr)
  T_fr/1 -> fr/1(T_fr)
  fr/1(w_fr) -> w_fr/1
  fl/1(w_fl) -> w_fl/1
  Fz_fl/1 -> fl/3(Fz_fl)
  Fx_fl/1 -> fl/2(Fx_fl)
  T_fl/1 -> fl/1(T_fl)

== system VMC_14Dof_2024a/Subsystem/alpha_lamda ==
  vx : Inport
  vy : Inport  Port=2
  wz : Inport  Port=3
  delta_fl : Inport  Port=4
  delta_fr : Inport  Port=5
  w_fl : Inport  Port=6
  w_fr : Inport  Port=7
  w_rl : Inport  Port=8
  w_rr : Inport  Port=9
  alpha : Subsystem
  lamda : Subsystem
  lamda_fl : Outport  VectorParamsAs1DForOutWhenUnconnected=off
  lamda_fr : Outport  Port=2  VectorParamsAs1DForOutWhenUnconnected=off
  lamda_rl : Outport  Port=3  VectorParamsAs1DForOutWhenUnconnected=off
  lamda_rr : Outport  Port=4  VectorParamsAs1DForOutWhenUnconnected=off
  alpha_fl : Outport  Port=5  VectorParamsAs1DForOutWhenUnconnected=off
  alpha_fr : Outport  Port=6  VectorParamsAs1DForOutWhenUnconnected=off
  alpha_rl : Outport  Port=7  VectorParamsAs1DForOutWhenUnconnected=off
  alpha_rr : Outport  Port=8  VectorParamsAs1DForOutWhenUnconnected=off
  wires:
  alpha/1(alpha_fl) -> alpha_fl/1
  alpha/2(alpha_fr) -> alpha_fr/1
  alpha/3(alpha_rl) -> alpha_rl/1
  alpha/4(alpha_rr) -> alpha_rr/1
  vx/1 -> lamda/1(vx), alpha/1(vx)
  vy/1 -> lamda/2(vy), alpha/2(vy)
  wz/1 -> lamda/3(wz), alpha/3(wz)
  delta_fl/1 -> lamda/4(delta_fl), alpha/4(delta_fl)
  delta_fr/1 -> lamda/5(delta_fr), alpha/5(delta_fr)
  w_fl/1 -> lamda/6(w_fl)
  w_fr/1 -> lamda/7(w_fr)
  w_rl/1 -> lamda/8(w_rl)
  w_rr/1 -> lamda/9(w_rr)
  lamda/1(lamda_fl) -> lamda_fl/1
  lamda/2(lamda_fr) -> lamda_fr/1
  lamda/4(lamda_rr) -> lamda_rr/1
  lamda/3(lamda_rl) -> lamda_rl/1

== system VMC_14Dof_2024a/Subsystem/rad//s_to_rpm ==
  w_fl : Inport
  w_fr : Inport  Port=2
  w_rl : Inport  Port=3
  w_rr : Inport  Port=4
  Gain{,1..3} (4 alike) : Gain  Gain=30/pi
  n_fl : Outport  VectorParamsAs1DForOutWhenUnconnected=off
  n_fr : Outport  Port=2  VectorParamsAs1DForOutWhenUnconnected=off
  n_rl : Outport  Port=3  VectorParamsAs1DForOutWhenUnconnected=off
  n_rr : Outport  Port=4  VectorParamsAs1DForOutWhenUnconnected=off
  wires:
  w_fl/1 -> Gain/1
  Gain/1 -> n_fl/1
  w_fr/1 -> Gain1/1
  w_rl/1 -> Gain2/1
  w_rr/1 -> Gain3/1
  Gain2/1 -> n_rl/1
  Gain1/1 -> n_fr/1
  Gain3/1 -> n_rr/1

== system VMC_14Dof_2024a/Subsystem1/Power_Limitation ==
  Cmd_Torque_Nm : Inport
  Vehicle_States_In : Inport  Port=2
  Controller_Setting : Inport  Port=3
  Bus Selector : BusSelector  OutputSignals=Power_Limitation.Tractive_Power_Limitation_kW,Power_Limitation.Regen_Power_Limitation_kW
  Bus Selector1 : BusSelector  OutputSignals=Power_Limitation.Tractive_Power_Limitation_kW,Power_Limitation.Regen_Power_Limitation_kW
  Bus Selector2 : BusSelector  OutputSignals=Accumulator.Power_kW
  FeedForward_PowerLimit : MATLAB Function  TreatAsAtomicUnit=on
  MATLAB Function : MATLAB Function  TreatAsAtomicUnit=on
  Power_Estimation : Subsystem
  Torque_out_Nm : Outport
  FF_PowerLimit_Factor_NA : Outport  Port=2
  wires:
  Vehicle_States_In/1 -> Bus Selector2/1, Power_Estimation/2(Vehicle_States_In)
  Cmd_Torque_Nm/1 -> Power_Estimation/1(Cmd_Torque_Nm), FeedForward_PowerLimit/1(Torque)
  Controller_Setting/1 -> Bus Selector1/1, Bus Selector/1
  Bus Selector/1 -> FeedForward_PowerLimit/3(Tractive_Limit_Power)  "<Tractive_Power_Limitation_kW>"
  Power_Estimation/1(Est_Power_kW) -> FeedForward_PowerLimit/2(Est_Power)  "Est_Power"
  Bus Selector/2 -> FeedForward_PowerLimit/4(Regen_Limit_Power)  "<Regen_Power_Limitation_kW>"
  FeedForward_PowerLimit/2(Torque_out) -> MATLAB Function/1(Torque)
  Bus Selector1/1 -> MATLAB Function/2(Tractive_Limit_Power)  "<Tractive_Power_Limitation_kW>"
  Bus Selector1/2 -> MATLAB Function/3(Regen_Limit_Power)  "<Regen_Power_Limitation_kW>"
  Bus Selector2/1 -> MATLAB Function/4(Act_Power)  "<Power_kW>"
  MATLAB Function/1(Torque_out) -> Torque_out_Nm/1
  FeedForward_PowerLimit/1(factor) -> FF_PowerLimit_Factor_NA/1

== system VMC_14Dof_2024a/Subsystem1/Subsystem ==
  TV_P : Inport
  TV_I : Inport  Port=2
  TV_D : Inport  Port=3
  TV_FF_Enable_bool : Inport  Port=4  OutDataTypeStr=boolean
  TV_FB_Enable_bool : Inport  Port=5  OutDataTypeStr=boolean
  TV_ExtMz_Sat_Nm : Inport  Port=6
  TV_ExtMz_Rate_Nmps : Inport  Port=7
  TC_P : Inport  Port=8
  TC_I : Inport  Port=9
  TC_D : Inport  Port=10
  Road_Coefficient_NA : Inport  Port=11
  TC_Enable_bool : Inport  Port=12
  Tractive_Power_Limitation_kW : Inport  Port=13
  Regen_Power_Limitation_kW : Inport  Port=14
  Bus Creator{,2..4} (4 alike) : BusCreator  Inputs=3
  Bus Creator1 : BusCreator  Inputs=5
  Bus Creator5 : BusCreator  Inputs=2
  Controller_Setting : Outport
  wires:
  TV_P/1 -> Bus Creator/1  "TV_P"
  TV_I/1 -> Bus Creator/2  "TV_I"
  TV_D/1 -> Bus Creator/3  "TV_D"
  Bus Creator/1 -> Bus Creator1/1  "TV_PID"
  TV_FF_Enable_bool/1 -> Bus Creator1/2  "TV_FF_Enable_bool"
  TV_FB_Enable_bool/1 -> Bus Creator1/3  "TV_FB_Enable_bool"
  TV_ExtMz_Sat_Nm/1 -> Bus Creator1/4  "TV_ExtMz_Sat_Nm"
  TV_ExtMz_Rate_Nmps/1 -> Bus Creator1/5  "TV_ExtMz_Rate_Nmps"
  TC_P/1 -> Bus Creator2/1  "TC_P"
  TC_I/1 -> Bus Creator2/2  "TC_I"
  TC_D/1 -> Bus Creator2/3  "TC_D"
  Bus Creator2/1 -> Bus Creator3/1  "TC_PID"
  Bus Creator1/1 -> Bus Creator4/1  "TV_Controller"
  Bus Creator3/1 -> Bus Creator4/2  "TC_Controller"
  Bus Creator4/1 -> Controller_Setting/1
  Road_Coefficient_NA/1 -> Bus Creator3/2  "Road_Coefficient_NA"
  TC_Enable_bool/1 -> Bus Creator3/3  "TC_Enable_bool"
  Bus Creator5/1 -> Bus Creator4/3  "Power_Limitation"
  Tractive_Power_Limitation_kW/1 -> Bus Creator5/1  "Tractive_Power_Limitation_kW"
  Regen_Power_Limitation_kW/1 -> Bus Creator5/2  "Regen_Power_Limitation_kW"
